simulink model "counter_compare"  (R2016a)
settings: Solver=FixedStepDiscrete  StartTime=0.0  StopTime=1000  FixedStep=1  RelTol=1e-3
libraries: hdlsllib x1
settings Model: Creator=duyvu  LastModifiedBy=duyvu

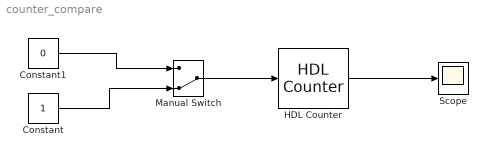
== system counter_compare ==
  Constant : Constant  OutDataTypeStr=boolean
  Constant1 : Constant  Value=0  OutDataTypeStr=boolean
  HDL Counter : hdlsllib/HDL Operations/HDL Counter  CountType=Free running  CountInit=0  CountStep=1  CountMax=25  CountFromType=Initial value  CountFrom=0  CountResetPort=off  CountLoadPort=off  CountEnbPort=on  CountDirPort=off  CountDataType=Unsigned  CountWordLen=8  CountFracLen=0  CountSampTime=1
  Manual Switch : ManualSwitch  CurrentSetting=0
  Scope : Scope
  wires:
  Constant1/1 -> Manual Switch/1
  Constant/1 -> Manual Switch/2
  Manual Switch/1 -> HDL Counter/1
  HDL Counter/1 -> Scope/1
